simulink library "constraints"  (Simulink 5.0)
libraries: simulink3 x2, simulink x1
settings Model: Creator=rlang  LastModifiedBy=rlang

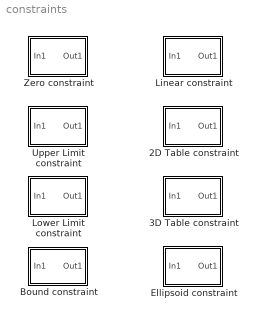
== system constraints ==
  2D Table constraint : Subsystem  mask(2D Table Constraints){NVar=4, InVar=1, OutVar=2, TabBrk=[-1 -0.5 0 0.5 1], TabVal=[1 1 1 .9 .7], Ineq=<=}
      mask prompts: NVar "Number of Variables:"; InVar "Input Variable:"; OutVar "Output Variable:"; TabBrk "Table Breakpoints:"; TabVal "Table Values:"; Ineq "Inequality:"
      mask help: This block implements 2D Table constraints for designs created in MBC.
      mask init:
      | % convert inequality to 1/-1 in Gain
      | Ineqval=2*(strmatch(Ineq,{'<=','>='},'exact')-1)-1;
      mask StyleString: edit,edit,edit,edit,edit,popup(<=|>=)
  3D Table constraint : Subsystem  mask(3D Table Constraints){NVar=4, InVarX=1, InVarY=2, OutVar=3, TabBrkX=[-1 -0 1], TabBrkY=[-1 0 1], TabVal=[1 1 1;1 1 .9;1 .9 .7], Ineq=<=}
      mask prompts: NVar "Number of Variables:"; InVarX "Input X Variable:"; InVarY "Input Y Variable:"; OutVar "Output Variable:"; TabBrkX "Table X breakpoints:"; TabBrkY "Table Y breakpoints:"; TabVal "Table Values"; Ineq "Inequality:"
      mask help: This block implements 3D Table constraints used in the MBC design objects.
      mask init:
      | % convert inequality to 1/-1 in Gain
      | Ineqval=2*(strmatch(Ineq,{'<=','>='},'exact')-1)-1;
      mask StyleString: edit,edit,edit,edit,edit,edit,edit,popup(<=|>=)
  Bound constraint : Subsystem  mask{B=}
  Ellipsoid constraint : Subsystem  mask(Ellipsoid Constraint){W=[1 0 0 0; 0 1 0 0; 0 0 1 0; 0 0 0 1], Xc=[0 0 0 0], SF=1}
      mask prompts: W "W Matrix:"; Xc "Offset vector:"; SF "Scale factor:"
      mask help: This block impements ellipsoid constraints for MBC design objects
  Linear constraint : Subsystem  mask(Linear Constraints){A=[1 1 1 1], b=.5}
      mask prompts: A "Linear coefficients:"; b "Inequality constant:"
      mask help: This block inplements Linear constraints for MBC design objects.
  Lower Limit constraint : Subsystem  mask(Lowe Bound Constraint){LB=[1 1 1 1]}
      mask prompts: LB "Upper bounds vector:"
      mask help: This block impements lower bound constraints for MBC design objects
  Upper Limit constraint : Subsystem  mask(Upper Bound Constraint){UB=[1 1 1 1]}
      mask prompts: UB "Upper bounds vector:"
      mask help: This block impements upper bound constraints for MBC design objects
  Zero constraint : Subsystem

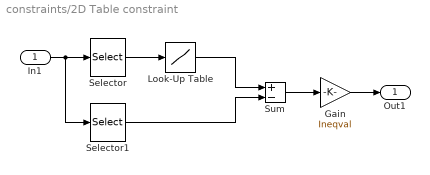
== system constraints/2D Table constraint ==
  In1 : Inport
  Gain : Gain  Gain=Ineqval  SaturateOnIntegerOverflow=on
  Look-Up Table : Lookup  InputValues=TabBrk  OutputValues=TabVal  SaturateOnIntegerOverflow=on
  Selector : Selector  Elements=InVar  InputPortWidth=NVar
  Selector1 : Selector  Elements=OutVar  InputPortWidth=NVar
  Sum : Sum  Inputs=+-  SaturateOnIntegerOverflow=on  InputSameDT=on
  Out1 : Outport
  wires:
  Selector1/1 -> Sum/2
  Look-Up Table/1 -> Sum/1
  Selector/1 -> Look-Up Table/1
  In1/1 -> Selector1/1, Selector/1
  Sum/1 -> Gain/1
  Gain/1 -> Out1/1

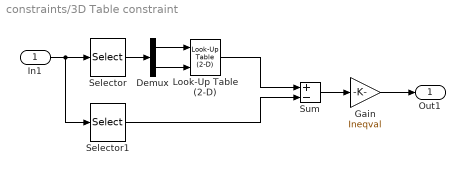
== system constraints/3D Table constraint ==
  In1 : Inport
  Demux : Demux  Outputs=2
  Gain : Gain  Gain=Ineqval  SaturateOnIntegerOverflow=on
  Look-Up Table (2-D) : simulink3/Functions & Tables/Look-Up Table (2-D)  x=TabBrkY  y=TabBrkX  t=TabVal  SettingsModeFixpt=off  LookUpMeth=Interpolation-Extrapolation  OutputDataTypeScalingMode=All ports same datatype  OutDataType=sfix(16)  OutScaling=2^-10  DoSatur=off  DblOver=off  dolog=off
  Selector : Selector  Elements=[InVarY InVarX]  InputPortWidth=NVar
  Selector1 : Selector  Elements=OutVar  InputPortWidth=NVar
  Sum : Sum  Inputs=+-  SaturateOnIntegerOverflow=on  InputSameDT=on
  Out1 : Outport
  wires:
  Look-Up Table (2-D)/1 -> Sum/1
  Selector1/1 -> Sum/2
  Selector/1 -> Demux/1
  Demux/2 -> Look-Up Table (2-D)/2
  Demux/1 -> Look-Up Table (2-D)/1
  In1/1 -> Selector/1, Selector1/1
  Sum/1 -> Gain/1
  Gain/1 -> Out1/1

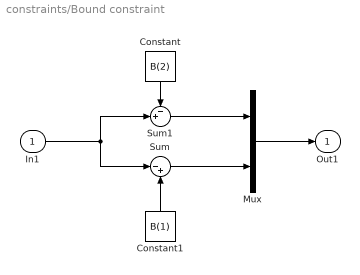
== system constraints/Bound constraint ==
  In1 : Inport
  Constant : Constant  Orientation=down  Value=B(2)
  Constant1 : Constant  Orientation=up  Value=B(1)
  Mux : Mux  Inputs=2
  Sum : Sum  Inputs=|-+  SaturateOnIntegerOverflow=on  InputSameDT=on
  Sum1 : Sum  Inputs=-+|  SaturateOnIntegerOverflow=on  InputSameDT=on
  Out1 : Outport
  wires:
  Constant1/1 -> Sum/2
  Constant/1 -> Sum1/1
  Mux/1 -> Out1/1
  Sum/1 -> Mux/2
  Sum1/1 -> Mux/1
  In1/1 -> Sum/1, Sum1/2

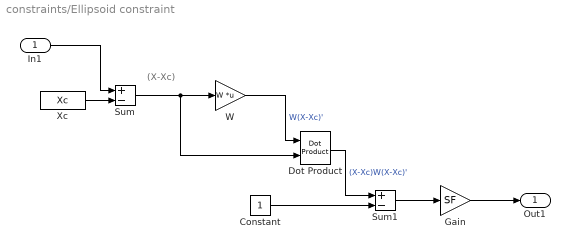
== system constraints/Ellipsoid constraint ==
  note: (X-Xc)
  In1 : Inport
  Constant : Constant
  Dot Product : simulink/Math Operations/Dot Product
  Gain : Gain  Gain=SF  SaturateOnIntegerOverflow=on
  Sum : Sum  Inputs=+-  SaturateOnIntegerOverflow=on  InputSameDT=on
  Sum1 : Sum  Inputs=+-  SaturateOnIntegerOverflow=on  InputSameDT=on
  W : Gain  Gain=W  Multiplication=Matrix(K*u)  SaturateOnIntegerOverflow=on
  Xc : Constant  Value=Xc
  Out1 : Outport
  wires:
  In1/1 -> Sum/1
  Xc/1 -> Sum/2
  W/1 -> Dot Product/1  "W(X-Xc)'"
  Sum/1 -> W/1, Dot Product/2
  Sum1/1 -> Gain/1
  Constant/1 -> Sum1/2
  Dot Product/1 -> Sum1/1  "(X-Xc)W(X-Xc)'"
  Gain/1 -> Out1/1

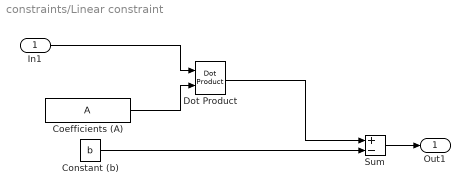
== system constraints/Linear constraint ==
  In1 : Inport
  Coefficients (A) : Constant  Value=A
  Constant (b) : Constant  Value=b
  Dot Product : simulink3/Math/Dot Product
  Sum : Sum  Inputs=+-  SaturateOnIntegerOverflow=on  InputSameDT=on
  Out1 : Outport
  wires:
  Constant (b)/1 -> Sum/2
  Sum/1 -> Out1/1
  Coefficients (A)/1 -> Dot Product/2
  In1/1 -> Dot Product/1
  Dot Product/1 -> Sum/1

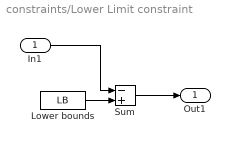
== system constraints/Lower Limit constraint ==
  In1 : Inport
  Lower bounds : Constant  Value=LB
  Sum : Sum  Inputs=-+  SaturateOnIntegerOverflow=on  InputSameDT=on
  Out1 : Outport
  wires:
  Sum/1 -> Out1/1
  In1/1 -> Sum/1
  Lower bounds/1 -> Sum/2

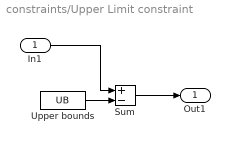
== system constraints/Upper Limit constraint ==
  In1 : Inport
  Sum : Sum  Inputs=+-  SaturateOnIntegerOverflow=on  InputSameDT=on
  Upper bounds : Constant  Value=UB
  Out1 : Outport
  wires:
  Upper bounds/1 -> Sum/2
  In1/1 -> Sum/1
  Sum/1 -> Out1/1

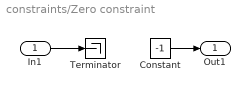
== system constraints/Zero constraint ==
  In1 : Inport
  Constant : Constant  Value=-1
  Terminator : Terminator
  Out1 : Outport
  wires:
  In1/1 -> Terminator/1
  Constant/1 -> Out1/1
